simulink model "H3DOF"  (R2023a)
settings: Solver=VariableStepAuto  StartTime=0.0  StopTime=10.0  RelTol=1e-3
libraries: simulink_extras x1
settings Model: Creator=jimmy  LastModifiedBy=jimmy

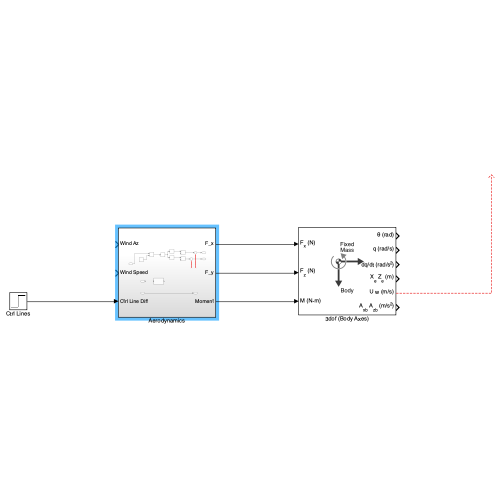
[thumbnail: Simulink's stored preview of the top-level diagram]
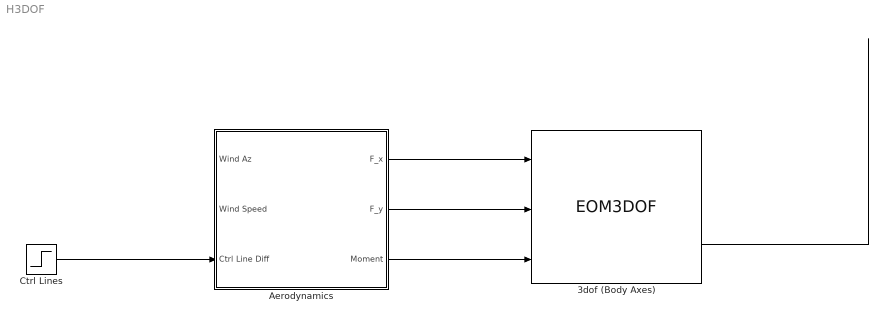
== system H3DOF ==
  3dof (Body Axes) : EOM3DOF  v_ini=2  theta_ini=45  q_ini=1  pos_ini=[-20 50]  mass=75  Iyy=200  vel_statename={'v_x', 'v_y'}  pos_statename={'x', 'y'}  q_statename='omega'  theta_statename='theta'
  Aerodynamics : Subsystem
  Ctrl Lines : Step  Before=1  After=2  SampleTime=0
  wires:
  Aerodynamics/3(Moment) -> 3dof (Body Axes)/3
  Aerodynamics/1(F_x) -> 3dof (Body Axes)/1
  Aerodynamics/2(F_y) -> 3dof (Body Axes)/2
  Ctrl Lines/1 -> Aerodynamics/3(Ctrl Line Diff)
  3dof (Body Axes)/5 -> ?

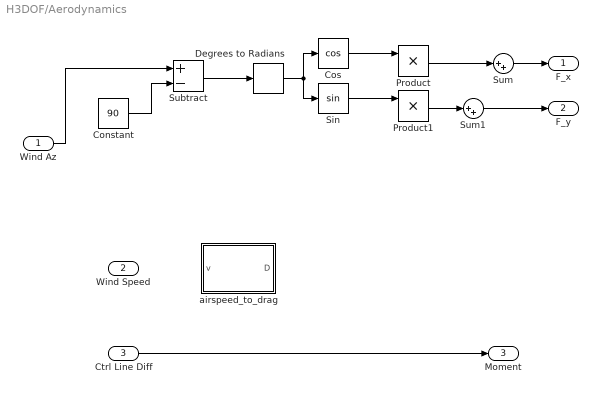
== system H3DOF/Aerodynamics ==
  Wind Az : Inport
  Wind Speed : Inport  Port=2
  Ctrl Line Diff : Inport  Port=3
  Constant : Constant  Value=90
  Cos : Trigonometry  Operator=cos
  Degrees to Radians : simulink_extras/Transformations/Degrees to Radians
  Product : Product
  Product1 : Product
  Sin : Trigonometry
  Subtract : Sum  Inputs=+-
  Sum : Sum  Inputs=|++
  Sum1 : Sum  Inputs=|++
  airspeed_to_drag : MATLAB Function  TreatAsAtomicUnit=on
  F_x : Outport
  F_y : Outport  Port=2
  Moment : Outport  Port=3
  wires:
  Ctrl Line Diff/1 -> Moment/1
  Wind Az/1 -> Subtract/1
  Degrees to Radians/1 -> Cos/1, Sin/1
  Cos/1 -> Product/1
  Sin/1 -> Product1/1
  Product/1 -> Sum/1
  Sum/1 -> F_x/1
  Product1/1 -> Sum1/1
  Sum1/1 -> F_y/1
  ? -> Sum1/2
  ? -> Sum/2
  Subtract/1 -> Degrees to Radians/1
  Constant/1 -> Subtract/2

== matlab function H3DOF/Aerodynamics/airspeed_to_drag ==
  data: v input; D output
function D = fcn(v)
% D: drag (N)
% v: airspeed (m/s)



% q: dynamic pressure (Pa)
% rho: 

C_d = 0.2;  % coefficient of drag
S = 2;      % projected area of the glider (m^2)
rho = 1.25; % air density at sea level (kg/m^3)

q = 0.5 * rho * v^2; % dynamic pressure


drag = C_d * q * S;
